simulink model "GFLIB_Sign_BAM_FLT"  (Simulink 7.3)
settings: Solver=ode45  StartTime=0.0  StopTime=10.0  RelTol=1e-3
settings Model: Creator=B17364  LastModifiedBy=B17364

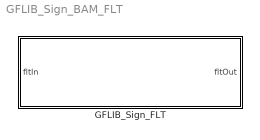
== system GFLIB_Sign_BAM_FLT ==
  GFLIB_Sign_FLT : Subsystem  mask(GFLIB_Sign_FLT){}
      mask help: Bit accurate model of the GFLIB_Sign function.
      mask init:
      | pos = get_param(gcb, 'Position');width = pos(3) - pos(1); height = pos(4) - pos(2);tX=width/2;tY=height*0.9;
      mask Display: color('black');port_label('input',1,'fltIn');port_label('output',1,'fltOut');color('black');disp('GFLIB_Sign_FLT');color('blue');text(tX,tY, 'BAM', 'horizontalAlignment', 'center');

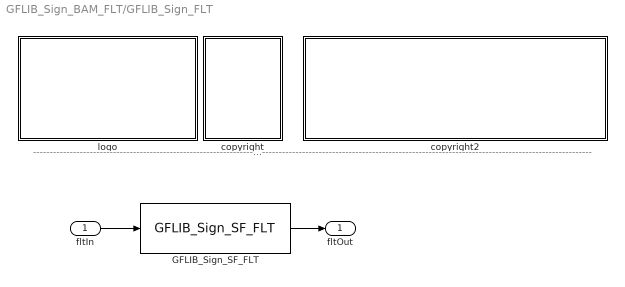
== system GFLIB_Sign_BAM_FLT/GFLIB_Sign_FLT ==
  note: ---------------------------------------------------------------------------------------------------------------------------------------------------------------------------------------------------
  fltIn : Inport  OutDataType=fixdt(1, 16)  OutScaling=2^0
  GFLIB_Sign_SF_FLT : S-Function  FunctionName=GFLIB_Sign_SF_FLT  EnableBusSupport=off
  copyright : Subsystem
      mask Display: text(10,90,'FILE:');text(10,75,'DESRIPTION:')text(10,60,'COPYRIGHT:')text(10,45,'VERSION:')text(10,30,'DATE:')
  copyright2 : Subsystem
      mask Display: text(10,90,'GFLIB_Sign_BAM_FLT.mdl');text(10,75,'Sign function.');text(10,60,'Freescale')text(10,45,'0.1');text(10,30,'26-Aug-2011');
  logo : Subsystem
      mask Display: image(imread('logo.jpg'))
  fltOut : Outport  OutDataType=fixdt(1, 16)  OutScaling=2^0
  wires:
  fltIn/1 -> GFLIB_Sign_SF_FLT/1
  GFLIB_Sign_SF_FLT/1 -> fltOut/1

== system GFLIB_Sign_BAM_FLT/GFLIB_Sign_FLT/copyright ==

== system GFLIB_Sign_BAM_FLT/GFLIB_Sign_FLT/copyright2 ==

== system GFLIB_Sign_BAM_FLT/GFLIB_Sign_FLT/logo ==
